simulink model "t1_block_diagram"  (R2024a)
settings: Solver=VariableStepAuto  StartTime=0.0  StopTime=10  RelTol=1e-3
model workspace (MATLAB code in the model file):
  | R=0.22;
  | K2=2.53*10^(-3); %Backconstans
  | C=7.72*10^(-7);
  | L=73*10^(-6);
  | J=1.3*10^(-5);
  | Kt=24.2*10^(-3); %Torque c
  | U=24;
  | TL = 0;%2635e-3;
  | reference_rpm_task3 = 12;
libraries: fl_lib x6, nesl_utility x4, slpidlib x1, ee_lib x1
settings Model: Creator=korvits  LastModifiedBy=korvits

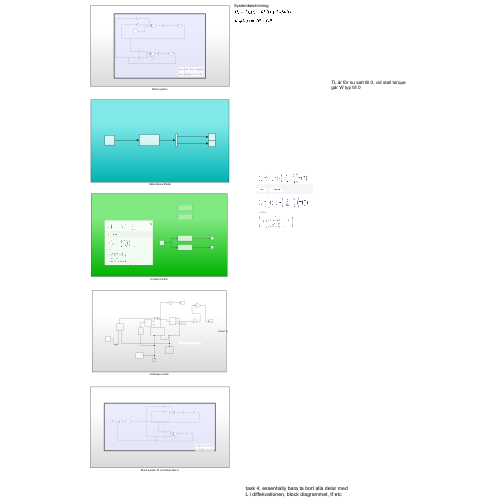
[thumbnail: Simulink's stored preview of the top-level diagram]
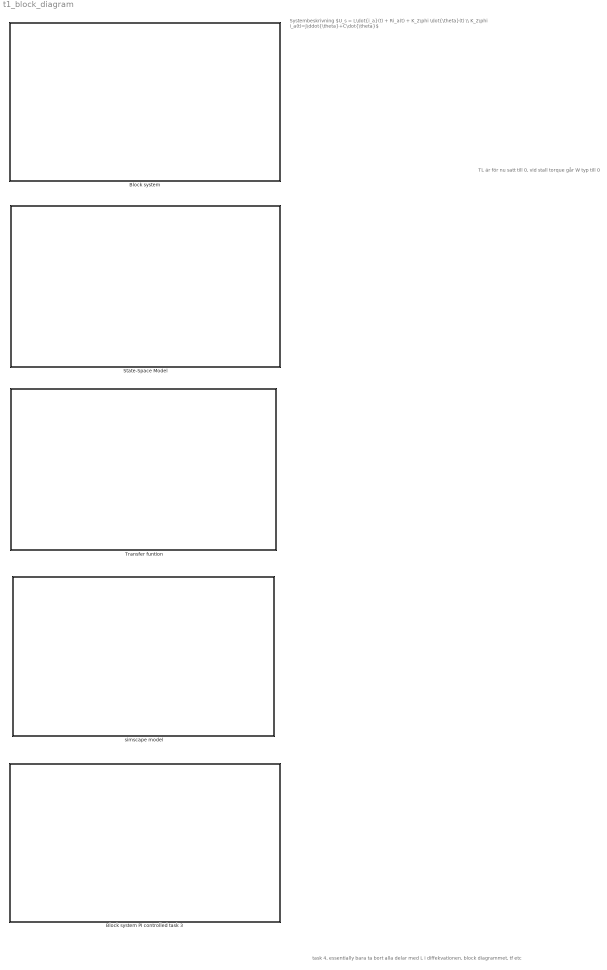
== system t1_block_diagram ==
  note: task 4, essentially bara ta bort alla delar med L i diffekvationen, block diagrammet, tf etc
  note: TL är för nu satt till 0, vid stall torque går W typ till 0
  note: Systembeskrivning
      | $U_s = L\dot{i_a}(t) + Ri_a(t) + K_2\phi \dot{\theta}(t) \\ K_2\phi i_a(t)=J\ddot{\theta}+C\dot{\theta}$
  Block system : Subsystem
  Block system PI controlled task 3 : Subsystem
  State-Space Model : Subsystem
  Transfer funtion : Subsystem
  simscape model : Subsystem

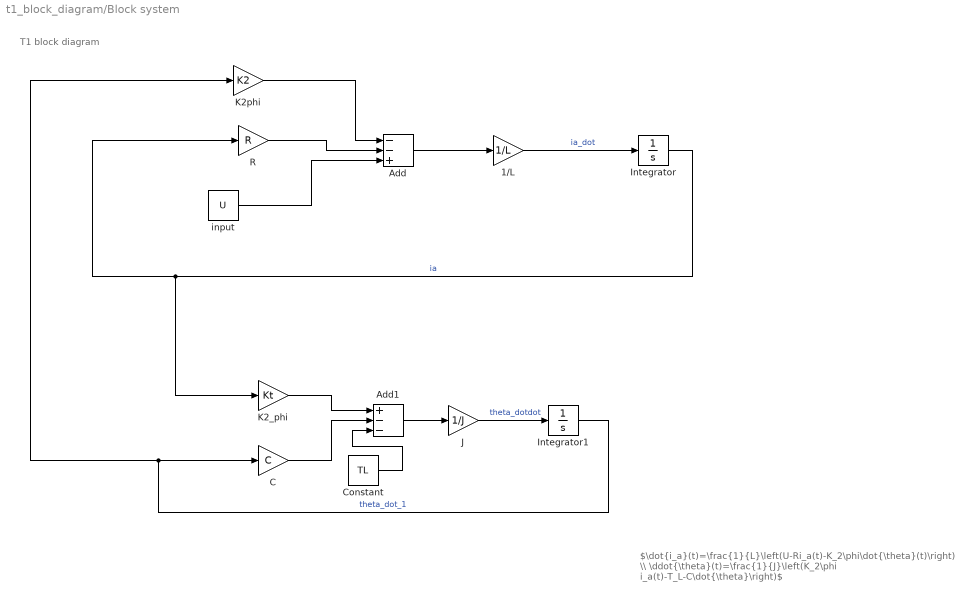
== system t1_block_diagram/Block system ==
  note: T1 block diagram
  note: $\dot{i_a}(t)=\frac{1}{L}\left(U-Ri_a(t)-K_2\phi\dot{\theta}(t)\right) \\ \ddot{\theta}(t)=\frac{1}{J}\left(K_2\phi i_a(t)-T_L-C\dot{\theta}\right)$
  1/L : Gain  Gain=1/L
  Add : Sum  Inputs=--+
  Add1 : Sum  Inputs=+--
  C : Gain  Gain=C
  Constant : Constant  Value=TL
  Integrator : Integrator
  Integrator1 : Integrator
  J : Gain  Gain=1/J
  K2_phi : Gain  Gain=Kt
  K2phi : Gain  Gain=K2
  R : Gain  Gain=R
  input : Constant  Value=U
  wires:
  R/1 -> Add/2
  K2_phi/1 -> Add1/1
  Add/1 -> 1/L/1
  1/L/1 -> Integrator/1  "ia_dot"
  K2phi/1 -> Add/1
  J/1 -> Integrator1/1  "theta_dotdot"
  input/1 -> Add/3
  Integrator/1 -> K2_phi/1, R/1  "ia"
  C/1 -> Add1/2
  Constant/1 -> Add1/3
  Integrator1/1 -> K2phi/1, C/1  "theta_dot_1"
  Add1/1 -> J/1

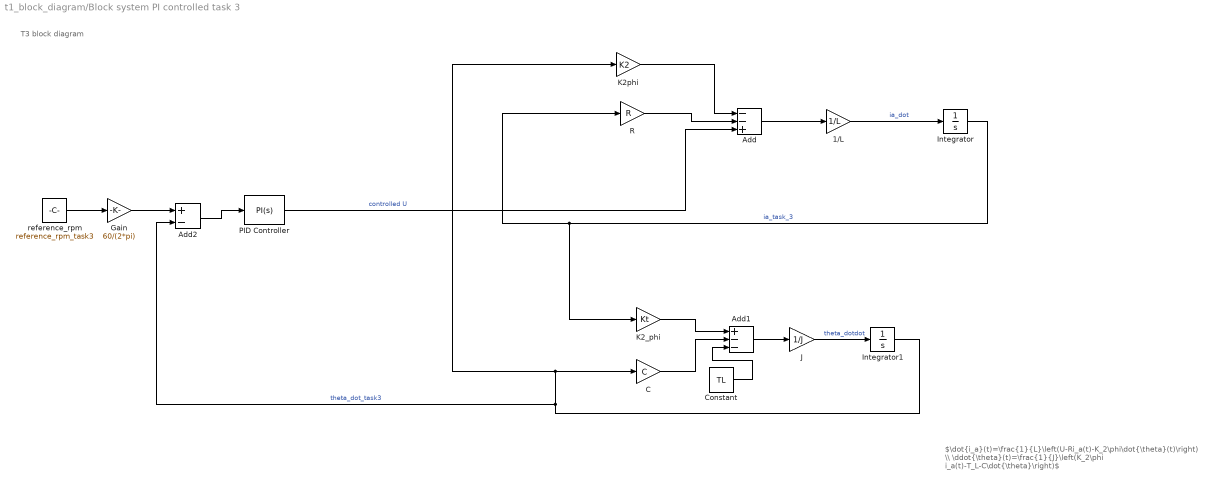
== system t1_block_diagram/Block system PI controlled task 3 ==
  note: T3 block diagram
  note: $\dot{i_a}(t)=\frac{1}{L}\left(U-Ri_a(t)-K_2\phi\dot{\theta}(t)\right) \\ \ddot{\theta}(t)=\frac{1}{J}\left(K_2\phi i_a(t)-T_L-C\dot{\theta}\right)$
  1/L : Gain  Gain=1/L
  Add : Sum  Inputs=--+
  Add1 : Sum  Inputs=+--
  Add2 : Sum  Inputs=+-
  C : Gain  Gain=C
  Constant : Constant  Value=TL
  Gain : Gain  Gain=60/(2*pi)
  Integrator : Integrator
  Integrator1 : Integrator
  J : Gain  Gain=1/J
  K2_phi : Gain  Gain=Kt
  K2phi : Gain  Gain=K2
  PID Controller : slpidlib/PID Controller  Controller=PI  Form=Parallel  TimeDomain=Continuous-time  UseExternalTs=off  SampleTime=-1  IntegratorMethod=Forward Euler  FilterMethod=Forward Euler  ControllerParametersSource=internal  P=0.0715720492726454  I=0.39217253662144  UseKiTs=off  D=0  UseExternalDerivativeSource=off  N=100  UseFilter=on  TunerSelectOption=Transfer Function Based (PID Tuner App)  InitialConditionSource=internal  InitialConditionForIntegrator=0  InitialConditionForFilter=0  DifferentiatorICPrevScaledInput=0  ExternalReset=none  TrackingMode=off  Kt=1  LimitOutput=off  SatLimitsSource=internal  UpperSaturationLimit=inf  LowerSaturationLimit=-inf  LinearizeAsGain=on  AntiWindupMode=none  Kb=1  LimitIntegrator=off  UpperIntegratorSaturationLimit=inf  LowerIntegratorSaturationLimit=-inf  POutMin=[]  POutMax=[]  IOutMin=[]  IOutMax=[]  DOutMin=[]  DOutMax=[]  NOutMin=[]  NOutMax=[]  SumOutMin=[]  SumOutMax=[]  SaturationOutMin=[]  SaturationOutMax=[]  PParamMin=[]  PParamMax=[]  IParamMin=[]  IParamMax=[]  DParamMin=[]  DParamMax=[]  NParamMin=[]  NParamMax=[]  KbParamMin=[]  KbParamMax=[]  KtParamMin=[]  KtParamMax=[]  KbOutMin=[]  KbOutMax=[]  KtOutMin=[]  KtOutMax=[]  IntegratorOutMin=[]  IntegratorOutMax=[]  FilterOutMin=[]  FilterOutMax=[]  SumI1OutMin=[]  SumI1OutMax=[]  SumI2OutMin=[]  SumI2OutMax=[]  SumI3OutMin=[]  SumI3OutMax=[]  SumI4OutMin=[]  SumI4OutMax=[]  SumDOutMin=[]  SumDOutMax=[]  DifferentiatorOutMin=[]  DifferentiatorOutMax=[]  FilterDiffOutCoefMin=[]  FilterDiffOutCoefMax=[]  ReciprocalOutMin=[]  ReciprocalOutMax=[]  SumDenOutMin=[]  SumDenOutMax=[]  SumNumOutMin=[]  SumNumOutMax=[]  DivideOutMin=[]  DivideOutMax=[]  UdiffTsProdOutMin=[]  UdiffTsProdOutMax=[]  NTsProdOutMin=[]  NTsProdOutMax=[]  UintegralTsProdOutMin=[]  UintegralTsProdOutMax=[]  UngainTsProdOutMin=[]  UngainTsProdOutMax=[]  ClampingZeroOutDataTypeStr=Inherit: Inherit via back propagation  ClampingZeroOutMin=[]  ClampingZeroOutMax=[]  FilterDenConstantOutDataTypeStr=Inherit: Inherit via back propagation  FilterDenConstantOutMin=[]  FilterDenConstantOutMax=[]  PCopyOutDataTypeStr=Inherit: Inherit via back propagation  PCopyOutMin=[]  PCopyOutMax=[]  NCopyOutDataTypeStr=Inherit: Inherit via back propagation  NCopyOutMin=[]  NCopyOutMax=[]  IntegratorContinuousStateAttributes=''  IntegratorStateMustResolveToSignalObject=off  IntegratorRTWStateStorageClass=Auto  FilterContinuousStateAttributes=''  FilterStateMustResolveToSignalObject=off  FilterRTWStateStorageClass=Auto  ParallelPVariant=InternalParameters  IdealPVariant=Disabled  IVariant=InternalParameters  DVariant=Disabled  IntegratorVariant=Continuous  SatVariant=Disabled  AWVariant=Passthrough  PCopyVariant=Disabled  TRVariant=Disabled  FdbkBlocksVariant=Forward  IdealPFdbkVariant=Disabled  SatFdbkVariant=Disabled  DerivativeFilterVariant=Disabled  NVariant=Disabled  NCopyVariant=Disabled_SignalSpec  FilterICVariant=Disabled  IntegratorICVariant=InternalICs  ExternalResetVariant=Disabled  TRSumVariant=Passthrough  SumFdbkVariant=Disabled  SumVariant=Sum_PI  TsampFilterVariant=InternalTs  TsampNgainVariant=Passthrough  TsampIntegralVariant=Disabled_SignalSpec  ExternalSaturationOutDataTypeStr=Inherit: Same as second input  DerivativeSourceVariant=Disabled
  R : Gain  Gain=R
  reference_rpm : Constant  Value=reference_rpm_task3
  wires:
  R/1 -> Add/2
  K2_phi/1 -> Add1/1
  Add/1 -> 1/L/1
  1/L/1 -> Integrator/1  "ia_dot"
  K2phi/1 -> Add/1
  J/1 -> Integrator1/1  "theta_dotdot"
  PID Controller/1 -> Add/3  "controlled U"
  Integrator/1 -> K2_phi/1, R/1  "ia_task_3"
  C/1 -> Add1/2
  Constant/1 -> Add1/3
  Integrator1/1 -> Add2/2, K2phi/1, C/1  "theta_dot_task3"
  Add1/1 -> J/1
  Add2/1 -> PID Controller/1
  reference_rpm/1 -> Gain/1
  Gain/1 -> Add2/1

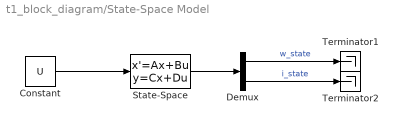
== system t1_block_diagram/State-Space Model ==
  Constant : Constant  Value=U
  Demux : Demux  Outputs=2
  State-Space : StateSpace  A=[-C/J, Kt/J; -K2/L, -R/L]  B=[-TL/(J*U); 1/L]  C=[1, 0; 0 1]  D=[0;0]  InitialCondition=0
  Terminator1 : Terminator
  Terminator2 : Terminator
  wires:
  Constant/1 -> State-Space/1
  State-Space/1 -> Demux/1
  Demux/2 -> Terminator2/1  "i_state"
  Demux/1 -> Terminator1/1  "w_state"

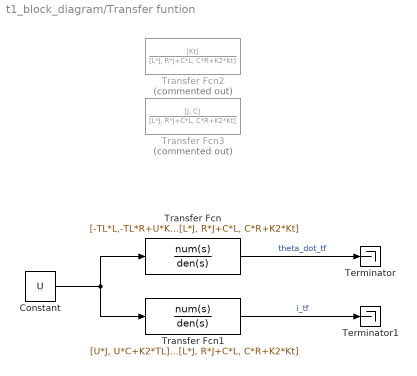
== system t1_block_diagram/Transfer funtion ==
  Constant : Constant  Value=U
  Terminator : Terminator
  Terminator1 : Terminator
  Transfer Fcn : TransferFcn  Numerator=[-TL*L,-TL*R+U*Kt]  Denominator=U.*[L*J, R*J+C*L, C*R+K2*Kt]
  Transfer Fcn1 : TransferFcn  Numerator=[U*J, U*C+K2*TL]  Denominator=U.*[L*J, R*J+C*L, C*R+K2*Kt]
  Transfer Fcn2 : TransferFcn  Commented=on  Numerator=[Kt]  Denominator=[L*J, R*J+C*L, C*R+K2*Kt]
  Transfer Fcn3 : TransferFcn  Commented=on  Numerator=[J, C]  Denominator=[L*J, R*J+C*L, C*R+K2*Kt]
  wires:
  Transfer Fcn1/1 -> Terminator1/1  "i_tf"
  Constant/1 -> Transfer Fcn1/1, Transfer Fcn/1
  Transfer Fcn/1 -> Terminator/1  "theta_dot_tf"

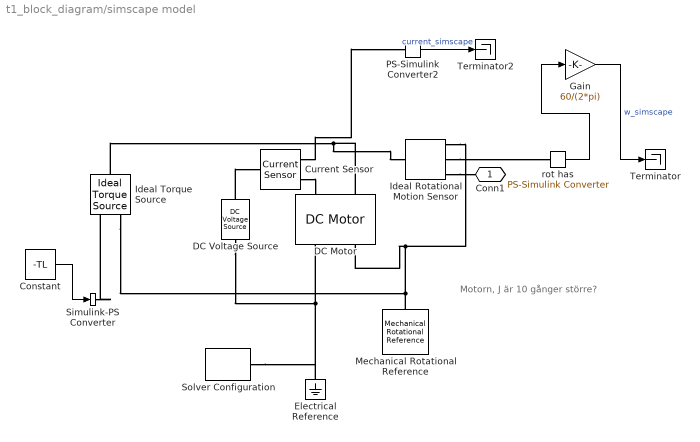
== system t1_block_diagram/simscape model ==
  note: Motorn, J är 10 gånger större?
  Constant : Constant  Value=-TL
  Current Sensor : fl_lib/Electrical/Electrical Sensors/Current Sensor
  DC Motor : ee_lib/Electromechanical/Brushed Motors/DC Motor  field_option=ee.enum.field_option.pm  Rf=100 Ohm  Lf=1 H  Laf=0.15 H  If0=0 A  parameterization=ee.enum.dcparam_option.circuit_param  Ra=R Ohm  La=L H  emf_or_torque=ee.enum.emf_or_torque.kv  Kv=K2 V/rpm  Ki=Kt N*m/A  T_stall=2635 mN*m  w_max=9700 rpm  w_rated=15000 rpm  P_rated=0.08 W  V_rated=24 V  lam_param=ee.enum.lam_param.damping  i_noload=0.527 A  V_i_noload=6 V  J=130*60/(2*pi) cm^2*g  lam=C N*m/(rpm)  speed0=0 rpm  enable_fault_armature=simscape.enum.onoff.off  rev_faulted=1 / 3  G_faulted_armature=1e-5 S  fault_trigger_armature=ee.enum.faults.faultTrigger.temporal  t_fault_armature=1 s  max_permissible_current_armature=inf A  t_fail_on_current_armature=1 s  enable_fault_field=simscape.enum.onoff.off  G_faulted_field=1e-5 S  fault_trigger_field=ee.enum.faults.faultTrigger.temporal  t_fault_field=1 s  max_permissible_current_field=inf A  t_fail_on_current_field=1 s  fault_action=simscape.enum.assert.action.none  alpha=3.93e-3 1/K  Tmeas=25 degC  thermal_mass=100 J/K  initial_temperature=25 degC
  DC Voltage Source : fl_lib/Electrical/Electrical Sources/DC Voltage Source  v0=U V
  Electrical Reference : fl_lib/Electrical/Electrical Elements/Electrical Reference
  Gain : Gain  Gain=60/(2*pi)
  Ideal Rotational Motion Sensor : fl_lib/Mechanical/Mechanical Sensors/Ideal Rotational Motion Sensor  reference=foundation.enum.MeasurementReference.difference  acceleration_port=false  velocity_port=true  position_port=true  wrap_angle=false  offset=0 rad
  Ideal Torque Source : fl_lib/Mechanical/Mechanical Sources/Ideal Torque Source
  Mechanical Rotational Reference : fl_lib/Mechanical/Rotational Elements/Mechanical Rotational Reference
  PS-Simulink Converter2 : nesl_utility/PS-Simulink Converter  PhysicalDomain=network_engine_domain  SubClassName=ps_output  LeftPortType=input  RightPortType=output  PseudoPeriodic=off  Frequencies=[]  VectorFormat=inherit  Unit=inherit  AffineConversion=off
  Simulink-PS Converter : nesl_utility/Simulink-PS Converter  PhysicalDomain=network_engine_domain  SubClassName=ps_input  LeftPortType=input  RightPortType=output  PseudoPeriodic=off  Frequencies=[]  NoiseDistribution=none  NoiseParameters=[]  Unit=1  AffineConversion=off  FilteringAndDerivatives=provide  SimscapeFilterOrder=1  InputFilterTimeConstant=0.001  UdotUserProvided=0
  Solver Configuration : nesl_utility/Solver Configuration  PhysicalDomain=network_engine_domain  SubClassName=solver  LeftPortType=input  RightPortType=generic  Tones=[]  Harmonics=[]  SimulateNoise=off  Profile=off  UseLocalSampling=off  EnableSwitchedLinearOptims=on  FrequencyDomain=off  UseCCode=off  RelTol=0.001  AbsTol=0.001  MinStep=1e-09  ToWorkspace=off  RevertToSquareIcSolve=off  NumHomotopyIterations=100  PhasorMode=off  PhasorModeNumHarmonics=1  ConsistencySolver=NEWTON_XTOL_AFTER_FTOL  IndexReductionMethod=DerivativeReplacement  DoDC=off  ResidualTolerance=1e-09  ConsistencyTolSource=GLOBAL  ConsistencyAbsTol=0.001  ConsistencyRelTol=0.001  ConsistencyTolFactor=0.001  UseLocalSolver=off  LocalSolverChoice=NE_BACKWARD_EULER_ADVANCER  ResolveIndetEquations=on  FunctionEvalNumThread=1  LocalSolverSampleTime=0.001  DoFixedCost=off  MaxNonlinIter=3  MaxModeIter=2  ComputeImpulses=off  ImpulseIterations=2  LinearAlgebra=auto  LinearAlgebraNumThread=0  EquationFormulation=NE_TIME_EF  DelaysMemoryBudget=1024  AutomaticFiltering=on  FilteringTimeConstant=0.001  PartitionStorageMethod=AS_NEEDED  PartitionMemoryBudget=1024  PartitionMethod=ROBUST  MultibodyUseLocalSolver=off  MultibodyLocalSolverChoice=ODE1  MultibodyLocalSolverSampleTime=0.001
  Terminator : Terminator
  Terminator2 : Terminator
  rot has : nesl_utility/PS-Simulink Converter  PhysicalDomain=network_engine_domain  SubClassName=ps_output  LeftPortType=input  RightPortType=output  PseudoPeriodic=off  Frequencies=[]  VectorFormat=inherit  Unit=inherit  AffineConversion=off
  Conn1 : PMIOPort  Side=Right
  wires:
  PS-Simulink Converter2/1 -> Terminator2/1  "current_simscape"
  Constant/1 -> Simulink-PS Converter/1
  rot has/1 -> Gain/1
  Gain/1 -> Terminator/1  "w_simscape"
  connections:
  Ideal Rotational Motion Sensor/RConn2 -- rot has/LConn1
  DC Voltage Source/LConn1 -- Current Sensor/LConn1
  Mechanical Rotational Reference/LConn1 -- Ideal Torque Source/RConn2 -- Ideal Rotational Motion Sensor/RConn1 -- DC Motor/RConn2
  DC Voltage Source/RConn1 -- Solver Configuration/RConn1 -- Electrical Reference/LConn1 -- DC Motor/RConn1
  Current Sensor/RConn1 -- PS-Simulink Converter2/LConn1
  Current Sensor/RConn2 -- DC Motor/LConn1
  Ideal Rotational Motion Sensor/RConn3 -- Conn1/RConn1
  Ideal Torque Source/LConn1 -- DC Motor/LConn2 -- Ideal Rotational Motion Sensor/LConn1
  Simulink-PS Converter/RConn1 -- Ideal Torque Source/RConn1
